simulink model "VIRTUAL_submition"  (R2025b)
settings: Solver=ode1  StartTime=0.0  StopTime=110  FixedStep=Controller_Sample_Time  RelTol=1e-3  EnableMultiTasking=on
values from neighbouring files (symbols this model uses):
  angles_qcar2 = angles_new_qcar2(2: length (angles_new_qcar2), width (angles_new_qcar2)-5)    [submit_script.m]
  cal_pos = [0, 0, 0]    [submit_script.m]
  Controller_Sample_Time = 1/500    (= 0.002)    [submit_script.m]
  CSI_Sample_Time = Controller_Sample_Time * ceil(0.033 / Controller_Sample_Time)    [submit_script.m]
  GyroKF_P0 = eye(2)    [submit_script.m]
  GyroKF_Q = diag([0.01, 0.001])    [submit_script.m]
  GyroKF_R = 0.01    [submit_script.m]
  GyroKF_X0 = [0;0]    [submit_script.m]
  ImageDisplay_Sample_Time = Controller_Sample_Time * 50    (= 0.1)    [submit_script.m]
  Initialization_Time = 5    [submit_script.m]
  LiDAR_Sample_Time = Controller_Sample_Time * ceil(1/15 / Controller_Sample_Time)    [submit_script.m]
  path_x4 = [repmat(hub(1), stop_len, 1); seg1(:,1); repmat(pickup(1), stop_len, 1);             seg2(:,1); seg3(:,1); repmat(dropoff(1), stop_len, 1);             seg4(:,1); repmat(hub(1), stop_len, 1)]    [submit_script.m]
  path_y4 = [repmat(hub(2), stop_len, 1); seg1(:,2); repmat(pickup(2), stop_len, 1);             seg2(:,2); seg3(:,2); repmat(dropoff(2), stop_len, 1);             seg4(:,2); repmat(hub(2), stop_len, 1)]    [submit_script.m]
  qcar2_lidar_to_map_rotation = 0    [submit_script.m]
  QCarEKF_L = 0.24    [submit_script.m]
  QCarEKF_P0 = eye(3)    [submit_script.m]
  QCarEKF_Q = diag([0.00001, 0.00001, 0.00001])    [submit_script.m]
  QCarEKF_R_combined = diag([0.1, 0.1, 0.01])    [submit_script.m]
  QCarEKF_R_heading = diag(0.1)    [submit_script.m]
  QcarKF_X0 = [0; 0; 0]    [submit_script.m]
  range_qcar2 = distance_new_qcar2(2: length (distance_new_qcar2), width (distance_new_qcar2)-5)    [submit_script.m]
  RealSense_Sample_Time = Controller_Sample_Time * ceil(0.033 / Controller_Sample_Time)    [submit_script.m]
undefined symbols (not defined in the file or in its folder): AAAF5050, gcbh, height, HIL, JPEG, K12, left, MC, Point, qc_get_step_size, top, video_display_show, width
libraries: quarc_library x42, simulink x3, simulink_extras x3
(part 3 of 3)

== matlab function VIRTUAL_submition/pathPlanner/Path 4  Look Ahead Generator/Windowed Closest Point Locator *Feedback the location1 ==
  data: x input; location output; y input; x_array input; y_array input; window input; global_search input; distance output; previous_location input
function [location,distance] = find_closest_window_point(x,y,x_array,y_array, window, global_search, previous_location)
distance = 1e6;
location = previous_location;
array_length = length (x_array);

if (global_search == 1)
    
    %Search the whole array (usually at startup)
    for i =1:array_length
        d = (x-x_array(i))^2 + (y-y_array(i))^2;
        if d < distance
            distance = d;
            location = i;
        end
    end
    
else
    
    if (location + window) > array_length
        %We need to wrap from the end
        % loop one - end of array:
        for i = (location-window):array_length
            d = (x-x_array(i))^2 + (y-y_array(i))^2;
            if d < distance
                distance = d;
                location = i;
            end
        end
        % loop two - start of array:
        for i = 1:(location+window-array_length)
            d = (x-x_array(i))^2 + (y-y_array(i))^2;
            if d < distance
                distance = d;
                location = i;
            end
        end
        
    elseif (location-window) < 1
        %We need to wrap from the beginning
        % loop one - end of array:
        for i = (array_length+location-window):array_length
            d = (x-x_array(i))^2 + (y-y_array(i))^2;
            if d < distance
                distance = d;
                location = i;
            end
        end
        % loop two - start of array:
        for i = 1:(location+window)
            d = (x-x_array(i))^2 + (y-y_array(i))^2;
            if d < distance
                distance = d;
                location = i;
            end
        end
        
    else
        %no need to wrap
        for i = (location-window):(location+window)
            d = (x-x_array(i))^2 + (y-y_array(i))^2;
            if d < distance
                distance = d;
                location = i;
            end
        end
    end
    
end
distance = sqrt(distance);
end

== matlab function VIRTUAL_submition/MATLAB Function ==
  settings: updateMethod=DISCRETE
  data: pathState output int32 size=1; pathIdx input
% function pathState = StateMachine(pathIdx)
% function pathState = StateMachine(pathIdx) %#codegen
% 
% % -------- PARAMETERS --------
% WAIT_TIME = 8;      % seconds
% Ts = 0.002;         % controller sample time
% 
% % -------- PERSISTENT MEMORY --------
% persistent startupCounter started
% if isempty(startupCounter)
%     startupCounter = int32(0);
%     started = false;
% end
% 
% % -------- SEGMENT LENGTHS --------
% seg1_len  = int32(2500);
% stop1_len = int32(500); %2000
% seg2_len  = int32(1500);
% stop2_len = int32(500); 
% seg3_len  = int32(1500);
% stop3_len = int32(500);
% 
% % -------- CUMULATIVE BOUNDS --------
% seg1_end  = seg1_len;
% stop1_end = seg1_end + stop1_len;
% seg2_end  = stop1_end + seg2_len;
% stop2_end = seg2_end + stop2_len;
% seg3_end  = stop2_end + seg3_len;
% stop3_end = seg3_end + stop3_len;
% 
% % -------- STARTUP WAIT (MAGENTA) --------
% if ~started
%     if startupCounter * Ts < WAIT_TIME
%         pathState = int32(6);      % MAGENTA – waiting
%         startupCounter = startupCounter + 1;
%         return
%     else
%         started = true;            % allow motion
%     end
% end
% 
% % -------- NORMAL PATH STATES --------
% if pathIdx <= seg1_end
%     pathState = int32(1);  % Driving to pickup
% elseif pathIdx <= stop1_end
%     pathState = int32(2);  % Pickup stop
% elseif pathIdx <= seg2_end
%     pathState = int32(3);  % Driving to dropoff
% elseif pathIdx <= stop2_end
%     pathState = int32(4);  % Dropoff stop
% elseif pathIdx <= seg3_end
%     pathState = int32(5);  % Returning to hub
% else
%     pathState = int32(6);  % Waiting at hub (magenta)
% end
% 
% % 1 = Driving to pickup
% % 2 = Pickup stop
% % 3 = Driving to dropoff
% % 4 = Dropoff stop
% % 5 = Driving to taxi hub
% % 6 = Waiting at hub

% function pathState = StateMachine(pathIdx) %#codegen
% % -------- PARAMETERS --------
% WAIT_TIME = 8;      % seconds
% Ts = 0.002;         % controller sample time
% 
% % -------- PERSISTENT MEMORY --------
% persistent startupCounter started
% if isempty(startupCounter)
%     startupCounter = int32(0);
%     started = false;
% end
% 
% % -------- VERIFIED LENGTHS FROM TRIAL 6 --------
% % These must match the path_x4 assembly exactly
% seg1_len  = int32(2500);  % Hub -> Pickup (P4)
% stop1_len = int32(5000);  % Pickup Stop (10s)
% seg2_len  = int32(1000);  % Pickup -> Junction (P4)
% seg3_len  = int32(1000);  % Junction -> Dropoff (P6 Left Turn)
% stop2_len = int32(5000);  % Dropoff Stop (10s)
% seg4_len  = int32(2500);  % Dropoff -> Hub (P6 Long Loop)
% % Note: Final stop is implicit (anything > seg4_end)
% 
% % -------- CUMULATIVE BOUNDS --------
% seg1_end  = seg1_len;
% stop1_end = seg1_end  + stop1_len;
% seg2_end  = stop1_end + seg2_len;
% seg3_end  = seg2_end  + seg3_len;
% stop2_end = seg3_end  + stop2_len;
% seg4_end  = stop2_end + seg4_len;
% 
% % -------- STARTUP WAIT (MAGENTA) --------
% if ~started
%     if cast(startupCounter, 'double') * Ts < WAIT_TIME
%         pathState = int32(7);      % Initial waiting state
%         startupCounter = startupCounter + 1;
%         return
%     else
%         started = true;            
%     end
% end
% 
% % -------- NORMAL PATH STATES --------
% if pathIdx <= seg1_end
%     pathState = int32(1);  % Driving to Pickup (Should work just like before)
% elseif pathIdx <= stop1_end
%     pathState = int32(2);  % Pickup Stop
% elseif pathIdx <= seg2_end
%     pathState = int32(3);  % Driving to Junction (Still on P4)
% elseif pathIdx <= seg3_end
%     pathState = int32(4);  % The Left Turn Switch (Now on P6)
% elseif pathIdx <= stop2_end
%     pathState = int32(5);  % Dropoff Stop
% elseif pathIdx <= seg4_end
%     pathState = int32(6);  % Long Return Loop (P6)
% else
%     pathState = int32(7);  % Final Stop at Hub
% end

% function pathState = StateMachine(pathIdx) %#codegen
% % -- 1. INITIALIZE OUTPUT (Fixes the 'Undefined' error) --
% pathState = int32(7); 
% 
% % -- 2. BOUNDARIES (Trial 33 - Total 30,000 pts) --
% % We use explicit integers to ensure type matching
% idx = int32(pathIdx);
% % 
% if idx <= 5000
%     pathState = int32(0);  % Initial Hub (Magenta)
% elseif idx <= 8000
%     pathState = int32(1);  % To Pickup (Green)
% elseif idx <= 13000
%     pathState = int32(2);  % Stop at Pickup (Blue)
% elseif idx <= 15000
%     pathState = int32(3);  % To Junction (Green)
% elseif idx <= 16000
%     pathState = int32(4);  % To Dropoff (Green)
% elseif idx <= 21000
%     pathState = int32(5);  % Stop at Dropoff (Orange)
% elseif idx <= 25000
%     pathState = int32(6);  % Return Loop (Green)
% else
%     pathState = int32(7);  % Final Hub Stop (Magenta)
% end
% % 
%In StateMachine Block:
% if idx <= 5000
%     pathState = int32(0); % Magenta Stop
% elseif idx <= 8000
%     pathState = int32(1); % Green Drive
% elseif idx <= 13000
%     pathState = int32(2); % Blue Stop
% elseif idx <= 15000
%     pathState = int32(3); % Green Drive
% elseif idx <= 16000
%     pathState = int32(4); % Green Drive 
% elseif idx <= 21000
%     pathState = int32(5); % ORANGE STOP 
% elseif idx <= 25000
%     pathState = int32(6); % Green Drive
% else
%     pathState = int32(7); % Magenta Final Stop
% end


%15
function pathState = StateMachine(pathIdx) %#codegen
    idx = int32(pathIdx);

WAIT_TIME = 8;      % seconds
Ts = 0.002;         % controller sample time

% -------- PERSISTENT MEMORY --------
persistent startupCounter started
if isempty(startupCounter)
    startupCounter = int32(0);
    started = false;
end

if ~started
    if cast(startupCounter, 'double') * Ts < WAIT_TIME
        pathState = int32(7);      % Initial waiting state
        startupCounter = startupCounter + 1;
        return
    else
        started = true;            
    end
end


    if idx <= 5000
        pathState = int32(0); % Hub Stop (Magenta)
    elseif idx <= 8000
        pathState = int32(1); % Drive to Pickup
    elseif idx <= 13000
        pathState = int32(2); % PICKUP STOP (Blue)
    elseif idx <= 16500
        pathState = int32(4); % Drive to Dropoff (Turning Left)
    elseif idx <= 21500
        pathState = int32(5); % --- DROPOFF STOP (Orange) ---
    elseif idx <= 25500
        pathState = int32(6); % Drive to Hub (Turning Right)
    else
        pathState = int32(7); % FINAL HUB STOP (Magenta)
    end
end

== matlab function VIRTUAL_submition/speedController/MATLAB Function ==
  settings: updateMethod=DISCRETE
  data: u input; y output; pathState input
%function y = fcn(u, pathState)
% 1 = Driving to pickup
% 2 = Pickup stop
% 3 = Driving to dropoff
% 4 = Dropoff stop
% 5 = Driving to taxi hub
% 6 = Waiting at hub

% function y = fcn(u, pathState)
% 
% % PARAMETERS
% WAIT_TIME = 8;      % seconds
% Ts = 0.002;         % controller sample time
% 
% % PERSISTENT MEMORY
% persistent stopCounter wasStopping
% if isempty(stopCounter)
%     stopCounter = 0;
%     wasStopping = false;
% end
% 
% % STOP STATES
% isStopState = (pathState == 2 || pathState == 5 || pathState == 7);
% 
% if isStopState
%     if ~wasStopping
%         % just entered stop state
%         stopCounter = 0;
%         wasStopping = true;
%     end
% 
%     if stopCounter * Ts < WAIT_TIME
%         y = 0;                 % keep stopped
%         stopCounter = stopCounter + 1;
%     else
%         y = u;                 % wait finished → move
%     end
% else
%     % normal driving
%     stopCounter = 0;
%     wasStopping = false;
%     y = u;
% end

% function y = fcn(u, pathState) %#codegen
% % -- 1. LOCK OUTPUT TYPE --
% y = 0.0; 
% 
% % -- 2. PARAMETERS --
% WAIT_TIME = 8.0;    
% Ts = 0.002;         
% 
% % -- 3. PERSISTENT MEMORY WITH FORCED TYPES --
% persistent stopCounter wasStopping lastState
% if isempty(stopCounter)
%     stopCounter = 0.0;
%     wasStopping = false;
%     % Using cast to ensure lastState is initialized as int32
%     lastState = cast(-1, 'int32'); 
% end
% 
% % -- 4. LOCAL TYPE ENFORCEMENT --
% % This line ensures the variable used in logic is definitely an int32
% current_state = int32(pathState);
% 
% % -- 5. IDENTIFY STOP STATES (Compare int32 to int32) --
% isStopState = (current_state == int32(0) || current_state == int32(2) || ...
%                current_state == int32(5) || current_state == int32(7));
% 
% % -- 6. RESET TIMER IF STATE CHANGES --
% if current_state ~= lastState
%     stopCounter = 0.0;
%     wasStopping = false;
% end
% 
% % Line 75: Both are now explicitly cast as int32
% lastState = current_state; 
% 
% % -- 7. STOPPING LOGIC --
% if isStopState
%     if ~wasStopping
%         stopCounter = 0.0;
%         wasStopping = true;
%     end
% 
%     if (stopCounter * Ts) < WAIT_TIME
%         y = 0.0; 
%         stopCounter = stopCounter + 1.0;
%     else
%         y = double(u); 
%     end
% else
%     stopCounter = 0.0;
%     wasStopping = false;
%     y = double(u);
% end

function y = fcn(u, pathState) %#codegen
% -- 1. LOCK OUTPUT TYPE --
y = 0.0; 

% -- 2. PERSISTENT MEMORY --
persistent stopCounter wasStopping lastState
if isempty(stopCounter)
    stopCounter = 0.0;
    wasStopping = false;
    lastState = int32(-1); % Explicitly cast to int32
end

% -- 3. PARAMETERS --
WAIT_TIME = 5.0;    % seconds
Ts = 0.002;         % controller sample time
current_s = int32(pathState);

% -- 4. IDENTIFY STOP STATES (0, 2, 5, 7) --
isStopState = (current_s == 0 || current_s == 2 || ...
               current_s == 5 || current_s == 7);

% -- 5. RESET TIMER IF STATE CHANGES --
if current_s ~= lastState
    stopCounter = 0.0;
    wasStopping = false;
end
lastState = current_s;

% -- 6. STOPPING LOGIC --
if isStopState
    if ~wasStopping
        stopCounter = 0.0;
        wasStopping = true;
    end
    
    if (stopCounter * Ts) < WAIT_TIME
        y = 0.0; % Stay stopped
        stopCounter = stopCounter + 1.0;
    else
        y = double(u); % Drive away
    end
else
    % Normal driving
    stopCounter = 0.0;
    wasStopping = false;
    y = double(u);
end

== matlab function VIRTUAL_submition/stateEstimation/Sensor Fusion - Complementary Filter/MATLAB Function ==
  data: car_speed input; correction_weight output; slope input; min_weight input
function correction_weight = weighting(car_speed, slope, min_weight)
correction_weight = 1 - 1*slope*car_speed;
if correction_weight < min_weight
    correction_weight = min_weight;
end
end

== matlab function VIRTUAL_submition/speedController/realsenseObstacleDetectionSpeedAdjust/MATLAB Function ==
  data: obstacle_distance input; speed_cmd output; stop_distance input; nominal_tracking_distance input; nominal_speed input
function speed_cmd = adaptive_cruise_control(obstacle_distance, stop_distance, nominal_tracking_distance, nominal_speed)

speed_cmd = nominal_speed;

if obstacle_distance < stop_distance
    speed_cmd = sat(nominal_speed,0,-1);
    
elseif obstacle_distance < nominal_tracking_distance
    speed_cmd = nominal_speed/(nominal_tracking_distance-stop_distance)*obstacle_distance...
        - nominal_speed/(nominal_tracking_distance-stop_distance)*stop_distance;
    
end

function output = sat (input, max,min)
if input > max
    output = max;
elseif input < min
    output = min;
else
    output = input;
end

== matlab function VIRTUAL_submition/obstacleDetection/obstacleDetection Markham March 22/Draw Lines Module ==
  data: img_in input; img_out output; pts input; color input
function img_out = drawLines(img_in, pts, color)

% Draw lines connecting the points using the provided color

% Inputs:
% u         : Input RGB Image (size = m by n)
% pts       : p x-y pairs of points (px) where markers are to be drawn
% color     : 1x3 matrix of RGB color values for each marker

% Outputs:
% y         : Output RGB Image with the markers drawn in (size = m by n)

%% Initialization
if size(img_in, 3) == 3
    img_out = img_in;
elseif size(img_in, 3) == 1
    img_out = cat(3, img_in, img_in, img_in);
end

[p, ~] = size(pts); % determine the number of points

%% Draw the lines
    for i = 1:p-1
        % determine the max(rows_difference, col_difference) between two
        % points
        itr = max(abs(pts(i,1) - pts(i+1,1)), abs(pts(i,2) - pts(i+1,2)));
        
        % generate linear spaces of row and col values between the pts
        row_vec = round(linspace(pts(i,1), pts(i+1,1), itr));
        col_vec = round(linspace(pts(i,2), pts(i+1,2), itr));
        
        % iterate through the values and shade them right

        for j = 1:itr
            img_out(row_vec(j), col_vec(j),1) = color(1);
            img_out(row_vec(j), col_vec(j),2) = color(2);
            img_out(row_vec(j), col_vec(j),3) = color(3);
        end
    end
end

== matlab function VIRTUAL_submition/obstacleDetection/obstacleDetection Markham March 22/Steering based image subselector ==
  data: pts output; depth input; distance output; steering input; minDistance input; maxDistance input; width input; height input; vertCenter input; maxSteering input; reduction input; maxSteeringWidth input
function [pts, distance] = estimateDepthInRegion(depth, steering, minDistance, maxDistance, width, height, vertCenter, maxSteering, reduction, maxSteeringWidth)
% Input: 640 x 360
[ROW, COL] = size(depth);
mark = COL/2 - (steering*(COL/2 - width/2)/maxSteering);
applied_width = max(width - abs(steering/maxSteeringWidth)*reduction*width, 60);
left_w = max(mark+1-(applied_width/2), 0); % pick the left end, but never let it get negative
right_w = min(left_w + applied_width, COL); % pick the right end, but never past the image width
upper_h = max(ROW*vertCenter-height/2+1, 0); % pick the upper end, but never let it get negative
lower_h = min(ROW*vertCenter+height/2, ROW); % pick the lower end, but never let it go past the image height
depth(:,1:40) = maxDistance; %this is to remove artifacts in the camera's left section
region = double(depth(upper_h:lower_h, left_w:right_w)); 
pts = [upper_h, left_w; upper_h, right_w; lower_h, right_w; lower_h, left_w; upper_h, left_w];
u_flat = reshape(region, 1, []);

temp = maxDistance*ones(1, length(u_flat));

for i = 1:length(u_flat)
    if (u_flat(i) >= minDistance) && (u_flat(i) <= maxDistance)
        temp(i) = u_flat(i);
    end
end

% u_flat(u_flat < minDistance) = [];
% u_flat(u_flat > maxDistance) = [];
% distance = mean(mean(u_flat));
distance = min(temp(:));
